simulink model "model_fully_coupled"  (R2021a)
settings: Solver=ode4  StartTime=0.0  StopTime=4  FixedStep=1e-2  RelTol=1e-3
values from neighbouring files (symbols this model uses):
  C_1 = [0.7887 -0.2113 -0.5774; -0.2113 0.7887 -0.5774; 0.5774 0.5774 0.5774]    [parameter.m]
  C_2 = [-0.2113 -0.5774 0.7887; 0.7887 -0.5774 -0.2113; 0.5774 0.5774 0.5774]    [parameter.m]
  C_3 = [-0.5774 0.7887 -0.2113; -0.5774 -0.2113 0.7887; 0.5774 0.5774 0.5774]    [parameter.m]
  d_1 = d    (= 4e-07)    [parameter.m]
  d_2 = d    (= 4e-07)    [parameter.m]
  d_3 = d    (= 4e-07)    [parameter.m]
  F = [0;0;0]    [parameter.m]
  g_s_1 = C_1(1:3,1)    [parameter.m]
  g_s_2 = C_2(1:3,1)    [parameter.m]
  g_s_3 = C_3(1:3,1)    [parameter.m]
  I = [1 0 0;0 1 0;0 0 1]    [parameter.m]
  I_hub_Bc = [550 0.1045 -0.0840; 0.1045 650 0.0001; -0.0840 0.0001 650]    [parameter.m]
  I_rw1_Wc1 = [1.5915E-4 0 1.54E-10; 0 0.8594E-4 0; 1.54E-10 0 0.8594E-4]    [parameter.m]
  I_rw1_Wc1_ = [0 -J_13_1 J_12_1; -J_13_1 (-2*J_23_1) (J_22_1-J_33_1); J_12_1 (J_22_1-J_33_1) (-2*J_23_1)]    [parameter.m]
  I_rw2_Wc2 = [1.5915E-4 0 1.54E-10; 0 0.8594E-4 0; 1.54E-10 0 0.8594E-4]    [parameter.m]
  I_rw2_Wc2_ = [0 -J_13_2 J_12_2; -J_13_2 (-2*J_23_2) (J_22_2-J_33_2); J_12_2 (J_22_2-J_33_2) (-2*J_23_2)]    [parameter.m]
  I_rw3_Wc3 = [1.5915E-4 0 1.54E-10; 0 0.8594E-4 0; 1.54E-10 0 0.8594E-4]    [parameter.m]
  I_rw3_Wc3_ = [0 -J_13_3 J_12_3; -J_13_3 (-2*J_23_3) (J_22_3-J_33_3); J_12_3 (J_22_3-J_33_3) (-2*J_23_3)]    [parameter.m]
  J_11_1 = I_rw1_Wc1(1,1)    [parameter.m]
  J_11_2 = I_rw2_Wc2(1,1)    [parameter.m]
  J_11_3 = I_rw3_Wc3(1,1)    [parameter.m]
  J_12_1 = I_rw1_Wc1(1,2)    [parameter.m]
  J_12_2 = I_rw2_Wc2(1,2)    [parameter.m]
  J_12_3 = I_rw3_Wc3(1,2)    [parameter.m]
  J_13_1 = I_rw1_Wc1(1,3)    [parameter.m]
  J_13_2 = I_rw2_Wc2(1,3)    [parameter.m]
  J_13_3 = I_rw3_Wc3(1,3)    [parameter.m]
  J_22_1 = I_rw1_Wc1(2,2)    [parameter.m]
  J_22_2 = I_rw2_Wc2(2,2)    [parameter.m]
  J_22_3 = I_rw3_Wc3(2,2)    [parameter.m]
  J_23_1 = I_rw1_Wc1(2,3)    [parameter.m]
  J_23_2 = I_rw2_Wc2(2,3)    [parameter.m]
  J_23_3 = I_rw3_Wc3(2,3)    [parameter.m]
  J_33_1 = I_rw1_Wc1(3,3)    [parameter.m]
  J_33_2 = I_rw2_Wc2(3,3)    [parameter.m]
  J_33_3 = I_rw3_Wc3(3,3)    [parameter.m]
  m_hub = 644    [parameter.m]
  m_rw_1 = m_rw(1)    [parameter.m]
  m_rw_2 = m_rw(2)    [parameter.m]
  m_rw_3 = m_rw(3)    [parameter.m]
  m_sc = 680    [parameter.m]
  OMEGA_1 = OMEGA(1)    [parameter.m]
  OMEGA_2 = OMEGA(2)    [parameter.m]
  OMEGA_3 = OMEGA(3)    [parameter.m]
  omega_BN = [omega ; omega; omega]    [parameter.m]
  r_Bc_B = [1e-2; -2e-2; 10e-2]    [parameter.m]
  r_BN = [0;0;0]    [parameter.m]
  r_W1_B = [0.6309; -0.1691; 0.4619]    [parameter.m]
  r_W2_B = [-0.1691; 0.6309; 0.4619]    [parameter.m]
  r_W3_B = [-0.4619; -0.4619; 0.4619]    [parameter.m]
  sigma_BN = [sigma; sigma; sigma]    [parameter.m]
  u_s_1 = u_s(1)    [parameter.m]
  u_s_2 = u_s(2)    [parameter.m]
  u_s_3 = u_s(3)    [parameter.m]
  w_2_1 = C_1(1:3,2)    [parameter.m]
  w_2_2 = C_2(1:3,2)    [parameter.m]
  w_2_3 = C_3(1:3,2)    [parameter.m]
  w_3_1 = C_1(1:3,3)    [parameter.m]
  w_3_2 = C_2(1:3,3)    [parameter.m]
  w_3_3 = C_3(1:3,3)    [parameter.m]
undefined symbols (not defined in the file or in its folder): deg, magnitude, rad, s
libraries: aerolibconvert2 x4, sharedutil x1, aerolibutil x1
(part 1 of 3)
settings Model: Creator=user  LastModifiedBy=user
settings DebuggingCC: AlgebraicLoopMsg=none

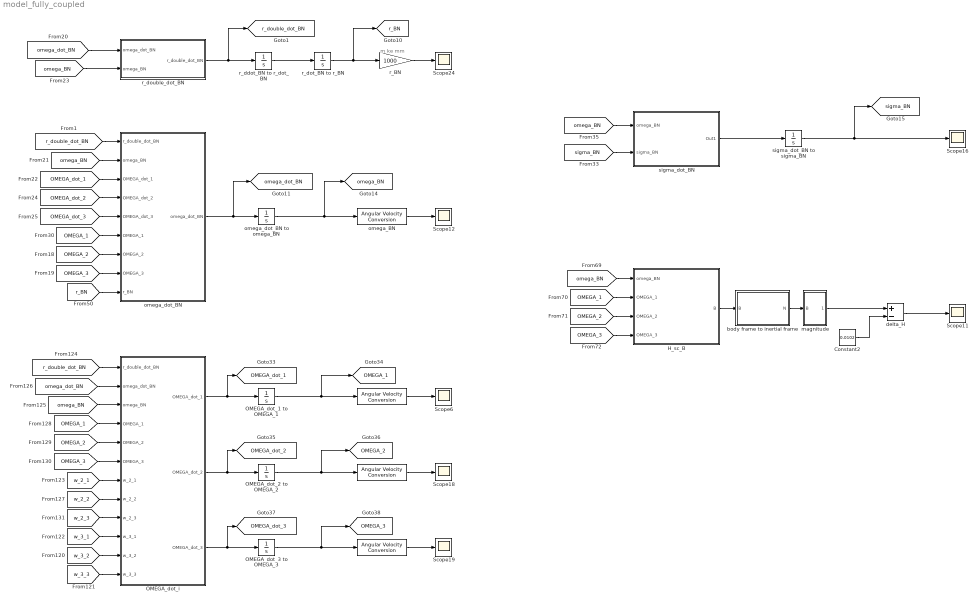
== system model_fully_coupled ==
  note: m ke mm
  " " : aerolibconvert2/Angular Velocity Conversion  IU=rad/s  OU=rpm
  "  " : aerolibconvert2/Angular Velocity Conversion  IU=rad/s  OU=rpm
  "   " : aerolibconvert2/Angular Velocity Conversion  IU=rad/s  OU=rpm
  Constant2 : Constant  Value=0.0102
  H_sc_B : Subsystem
  OMEGA_dot_1 to OMEGA_1 : Integrator  InitialCondition=OMEGA_1
  OMEGA_dot_2 to OMEGA_2 : Integrator  InitialCondition=OMEGA_2
  OMEGA_dot_3 to OMEGA_3 : Integrator  InitialCondition=OMEGA_3
  OMEGA_dot_i : Subsystem
  Scope{6,11..12,16,18..19,24} (7 alike) : Scope
  body frame to inertial frame : Subsystem
  delta_H : Sum  Inputs=+-
  magnitude : Subsystem
  omega_BN : aerolibconvert2/Angular Velocity Conversion  IU=rad/s  OU=deg/s
  omega_dot_BN : Subsystem
  omega_dot_BN to omega_BN : Integrator  InitialCondition=omega_BN
  r_BN : Gain  Gain=1000
  r_ddot_BN to r_dot_BN : Integrator  InitialCondition=r_BN
  r_dot_BN to r_BN : Integrator  InitialCondition=r_BN
  r_double_dot_BN : Subsystem
  sigma_dot_BN : Subsystem
  sigma_dot_BN to sigma_BN : Integrator  InitialCondition=sigma_BN
  tag scope: OMEGA_1=global, OMEGA_2=global, OMEGA_3=global, OMEGA_dot_1=global, OMEGA_dot_2=global, OMEGA_dot_3=global, omega_BN=global, omega_dot_BN=global, r_BN=global, r_double_dot_BN=global, sigma_BN=global
  wires:
  magnitude/1(Out1) -> delta_H/1
  [OMEGA_2] -> H_sc_B/3(OMEGA_2)
  H_sc_B/1(B) -> body frame to inertial frame/1(B)
  delta_H/1 -> Scope11/1
  [OMEGA_3] -> H_sc_B/4(OMEGA_3)
  [omega_BN] -> H_sc_B/1(omega_BN)
  [OMEGA_1] -> H_sc_B/2(OMEGA_1)
  Constant2/1 -> delta_H/2
  body frame to inertial frame/1(N) -> magnitude/1(B)
  r_dot_BN to r_BN/1 -> r_BN/1, [r_BN]
  r_double_dot_BN/1(r_double_dot_BN) -> [r_double_dot_BN], r_ddot_BN to r_dot_BN/1
  [omega_BN] -> r_double_dot_BN/2(omega_BN)
  r_ddot_BN to r_dot_BN/1 -> r_dot_BN to r_BN/1
  [omega_dot_BN] -> r_double_dot_BN/1(omega_dot_BN)
  r_BN/1 -> Scope24/1
  OMEGA_dot_2 to OMEGA_2/1 -> "  "/1, [OMEGA_2]
  [w_2_3] -> OMEGA_dot_i/9(w_2_3)
  [w_3_3] -> OMEGA_dot_i/12(w_3_3)
  [w_2_1] -> OMEGA_dot_i/7(w_2_1)
  OMEGA_dot_1 to OMEGA_1/1 -> [OMEGA_1], "   "/1
  [w_2_2] -> OMEGA_dot_i/8(w_2_2)
  OMEGA_dot_i/1(OMEGA_dot_1) -> OMEGA_dot_1 to OMEGA_1/1, [OMEGA_dot_1]
  [OMEGA_1] -> OMEGA_dot_i/4(OMEGA_1)
  OMEGA_dot_i/3(OMEGA_dot_3) -> [OMEGA_dot_3], OMEGA_dot_3 to OMEGA_3/1
  OMEGA_dot_i/2(OMEGA_dot_2) -> OMEGA_dot_2 to OMEGA_2/1, [OMEGA_dot_2]
  [omega_dot_BN] -> OMEGA_dot_i/2(omega_dot_BN)
  [omega_BN] -> OMEGA_dot_i/3(omega_BN)
  [r_double_dot_BN] -> OMEGA_dot_i/1(r_double_dot_BN)
  [OMEGA_2] -> OMEGA_dot_i/5(OMEGA_2)
  [w_3_2] -> OMEGA_dot_i/11(w_3_2)
  OMEGA_dot_3 to OMEGA_3/1 -> " "/1, [OMEGA_3]
  "   "/1 -> Scope6/1
  "  "/1 -> Scope18/1
  [w_3_1] -> OMEGA_dot_i/10(w_3_1)
  " "/1 -> Scope19/1
  [OMEGA_3] -> OMEGA_dot_i/6(OMEGA_3)
  [OMEGA_dot_2] -> omega_dot_BN/4(OMEGA_dot_2)
  omega_BN/1 -> Scope12/1
  omega_dot_BN to omega_BN/1 -> omega_BN/1, [omega_BN]
  [OMEGA_2] -> omega_dot_BN/7(OMEGA_2)
  [OMEGA_dot_3] -> omega_dot_BN/5(OMEGA_dot_3)
  [r_BN] -> omega_dot_BN/9(r_BN)
  [OMEGA_dot_1] -> omega_dot_BN/3(OMEGA_dot_1)
  [OMEGA_3] -> omega_dot_BN/8(OMEGA_3)
  [OMEGA_1] -> omega_dot_BN/6(OMEGA_1)
  omega_dot_BN/1("omega_dot_BN ") -> [omega_dot_BN], omega_dot_BN to omega_BN/1
  [omega_BN] -> omega_dot_BN/2(omega_BN)
  sigma_dot_BN/1(Out1) -> sigma_dot_BN to sigma_BN/1
  sigma_dot_BN to sigma_BN/1 -> Scope16/1, [sigma_BN]
  [sigma_BN] -> sigma_dot_BN/2(sigma_BN)
  [omega_BN] -> sigma_dot_BN/1(omega_BN)
  [r_double_dot_BN] -> omega_dot_BN/1(r_double_dot_BN)

== system model_fully_coupled/H_sc_B ==
  omega_BN : Inport
  OMEGA_1 : Inport  Port=2
  OMEGA_2 : Inport  Port=3
  OMEGA_3 : Inport  Port=4
  1 : Subsystem
  2 : Subsystem
  Add : Sum
  B : Outport
  wires:
  omega_BN/1 -> 2/1(omega_BN), 1/1(omega_BN)
  1/1(Out1) -> Add/1
  OMEGA_2/1 -> 2/3(OMEGA_2)
  OMEGA_3/1 -> 2/4(OMEGA_3)
  2/1(Out1) -> Add/2
  Add/1 -> B/1
  OMEGA_1/1 -> 2/2(OMEGA_1)

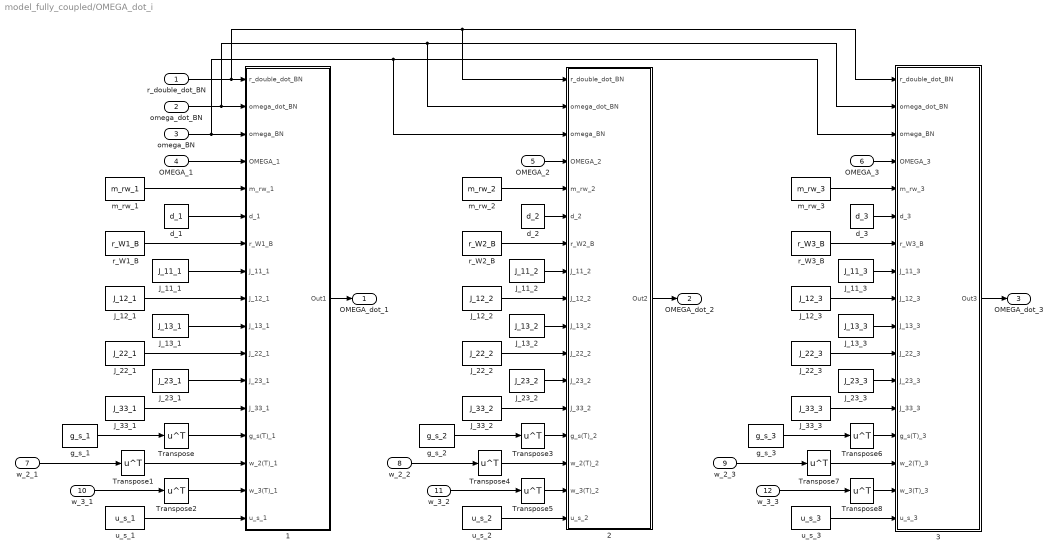
== system model_fully_coupled/OMEGA_dot_i ==
  r_double_dot_BN : Inport
  omega_dot_BN : Inport  Port=2
  omega_BN : Inport  Port=3
  OMEGA_1 : Inport  Port=4
  OMEGA_2 : Inport  Port=5
  OMEGA_3 : Inport  Port=6
  w_2_1 : Inport  Port=7
  w_2_2 : Inport  Port=8
  w_2_3 : Inport  Port=9
  w_3_1 : Inport  Port=10
  w_3_2 : Inport  Port=11
  w_3_3 : Inport  Port=12
  1 : Subsystem
  2 : Subsystem
  3 : Subsystem
  J_11_1 : Constant  Value=J_11_1
  J_11_2 : Constant  Value=J_11_2
  J_11_3 : Constant  Value=J_11_3
  J_12_1 : Constant  Value=J_12_1
  J_12_2 : Constant  Value=J_12_2
  J_12_3 : Constant  Value=J_12_3
  J_13_1 : Constant  Value=J_13_1
  J_13_2 : Constant  Value=J_13_2
  J_13_3 : Constant  Value=J_13_3
  J_22_1 : Constant  Value=J_22_1
  J_22_2 : Constant  Value=J_22_2
  J_22_3 : Constant  Value=J_22_3
  J_23_1 : Constant  Value=J_23_1
  J_23_2 : Constant  Value=J_23_2
  J_23_3 : Constant  Value=J_23_3
  J_33_1 : Constant  Value=J_33_1
  J_33_2 : Constant  Value=J_33_2
  J_33_3 : Constant  Value=J_33_3
  Transpose{,1..8} (9 alike) : Math  Operator=transpose  SaturateOnIntegerOverflow=on
  d_1 : Constant  Value=d_1
  d_2 : Constant  Value=d_2
  d_3 : Constant  Value=d_3
  g_s_1 : Constant  Value=g_s_1
  g_s_2 : Constant  Value=g_s_2
  g_s_3 : Constant  Value=g_s_3
  m_rw_1 : Constant  Value=m_rw_1
  m_rw_2 : Constant  Value=m_rw_2
  m_rw_3 : Constant  Value=m_rw_3
  r_W1_B : Constant  Value=r_W1_B
  r_W2_B : Constant  Value=r_W2_B
  r_W3_B : Constant  Value=r_W3_B
  u_s_1 : Constant  Value=u_s_1
  u_s_2 : Constant  Value=u_s_2
  u_s_3 : Constant  Value=u_s_3
  OMEGA_dot_1 : Outport
  OMEGA_dot_2 : Outport  Port=2
  OMEGA_dot_3 : Outport  Port=3
  wires:
  Transpose1/1 -> 1/15(w_2(T)_1)
  omega_dot_BN/1 -> 2/2(omega_dot_BN), 3/2(omega_dot_BN), 1/2(omega_dot_BN)
  w_3_1/1 -> Transpose2/1
  r_double_dot_BN/1 -> 2/1(r_double_dot_BN), 3/1(r_double_dot_BN), 1/1(r_double_dot_BN)
  g_s_1/1 -> Transpose/1
  J_23_1/1 -> 1/12(J_23_1)
  2/1(Out2) -> OMEGA_dot_2/1
  1/1(Out1) -> OMEGA_dot_1/1
  d_1/1 -> 1/6(d_1)
  m_rw_1/1 -> 1/5(m_rw_1)
  Transpose/1 -> 1/14(g_s(T)_1)
  J_33_1/1 -> 1/13(J_33_1)
  J_12_1/1 -> 1/9(J_12_1)
  omega_BN/1 -> 3/3(omega_BN), 2/3(omega_BN), 1/3(omega_BN)
  u_s_1/1 -> 1/17(u_s_1)
  Transpose2/1 -> 1/16(w_3(T)_1)
  3/1(Out3) -> OMEGA_dot_3/1
  J_11_1/1 -> 1/8(J_11_1)
  J_22_1/1 -> 1/11(J_22_1)
  J_13_1/1 -> 1/10(J_13_1)
  r_W1_B/1 -> 1/7(r_W1_B)
  w_2_1/1 -> Transpose1/1
  g_s_2/1 -> Transpose3/1
  J_23_2/1 -> 2/12(J_23_2)
  w_3_2/1 -> Transpose5/1
  r_W2_B/1 -> 2/7(r_W2_B)
  J_22_2/1 -> 2/11(J_22_2)
  J_11_2/1 -> 2/8(J_11_2)
  u_s_2/1 -> 2/17(u_s_2)
  J_12_2/1 -> 2/9(J_12_2)
  w_2_2/1 -> Transpose4/1
  Transpose3/1 -> 2/14(g_s(T)_2)
  m_rw_2/1 -> 2/5(m_rw_2)
  Transpose5/1 -> 2/16(w_3(T)_2)
  d_2/1 -> 2/6(d_2)
  J_33_2/1 -> 2/13(J_33_2)
  J_13_2/1 -> 2/10(J_13_2)
  Transpose4/1 -> 2/15(w_2(T)_2)
  g_s_3/1 -> Transpose6/1
  J_23_3/1 -> 3/12(J_23_3)
  w_3_3/1 -> Transpose8/1
  r_W3_B/1 -> 3/7(r_W3_B)
  J_22_3/1 -> 3/11(J_22_3)
  J_11_3/1 -> 3/8(J_11_3)
  u_s_3/1 -> 3/17(u_s_3)
  J_12_3/1 -> 3/9(J_12_3)
  w_2_3/1 -> Transpose7/1
  Transpose6/1 -> 3/14(g_s(T)_3)
  m_rw_3/1 -> 3/5(m_rw_3)
  Transpose8/1 -> 3/16(w_3(T)_3)
  d_3/1 -> 3/6(d_3)
  J_33_3/1 -> 3/13(J_33_3)
  J_13_3/1 -> 3/10(J_13_3)
  Transpose7/1 -> 3/15(w_2(T)_3)
  OMEGA_1/1 -> 1/4(OMEGA_1)
  OMEGA_2/1 -> 2/4(OMEGA_2)
  OMEGA_3/1 -> 3/4(OMEGA_3)

== system model_fully_coupled/body frame to inertial frame ==
  B : Inport
  MATLAB Function : MATLAB Function  TreatAsAtomicUnit=on
  N : Outport
  wires:
  MATLAB Function/1(N) -> N/1
  B/1 -> MATLAB Function/1(B)
  [sigma_BN] -> MATLAB Function/2(sigma_BN)

== system model_fully_coupled/magnitude ==
  B : Inport
  Add : Sum  Inputs=+++
  Demux : Demux  Outputs=3
  Magnitude Squared : Math  Operator=magnitude^2  SaturateOnIntegerOverflow=on
  Magnitude Squared1 : Math  Operator=magnitude^2  SaturateOnIntegerOverflow=on
  Magnitude Squared2 : Math  Operator=magnitude^2  SaturateOnIntegerOverflow=on
  Sqrt : Sqrt  SaturateOnIntegerOverflow=on
  Out1 : Outport
  wires:
  Add/1 -> Sqrt/1
  B/1 -> Demux/1
  Sqrt/1 -> Out1/1
  Demux/1 -> Magnitude Squared/1
  Demux/2 -> Magnitude Squared1/1
  Demux/3 -> Magnitude Squared2/1
  Magnitude Squared1/1 -> Add/2
  Magnitude Squared/1 -> Add/1
  Magnitude Squared2/1 -> Add/3

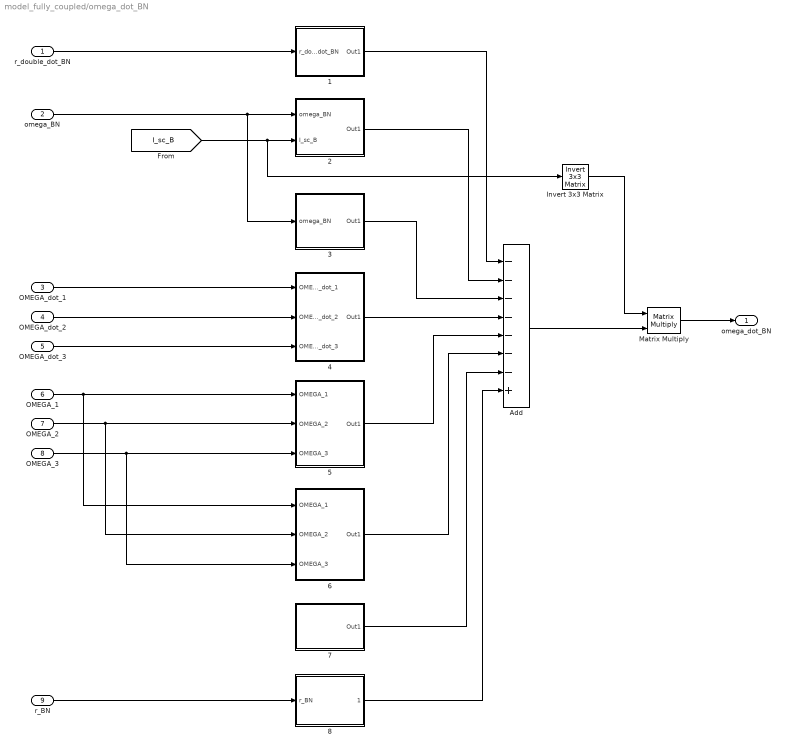
== system model_fully_coupled/omega_dot_BN ==
  r_double_dot_BN : Inport
  omega_BN : Inport  Port=2
  OMEGA_dot_1 : Inport  Port=3
  OMEGA_dot_2 : Inport  Port=4
  OMEGA_dot_3 : Inport  Port=5
  OMEGA_1 : Inport  Port=6
  OMEGA_2 : Inport  Port=7
  OMEGA_3 : Inport  Port=8
  r_BN : Inport  Port=9
  1 : Subsystem
  "2 " : Subsystem
  3 : Subsystem
  4 : Subsystem
  5 : Subsystem
  6 : Subsystem
  "7 " : Subsystem
  8 : Subsystem
  Add : Sum  Inputs=-------+
  Invert 3x3 Matrix : aerolibutil/Invert  3x3 Matrix
  Matrix Multiply : Product  Multiplication=Matrix(*)
  "omega_dot_BN " : Outport
  wires:
  OMEGA_2/1 -> 6/2(OMEGA_2), 5/2(OMEGA_2)
  OMEGA_dot_3/1 -> 4/3(OMEGA_dot_3)
  OMEGA_1/1 -> 6/1(OMEGA_1), 5/1(OMEGA_1)
  OMEGA_dot_1/1 -> 4/1(OMEGA_dot_1)
  omega_BN/1 -> 3/1(omega_BN), "2 "/1(omega_BN)
  OMEGA_dot_2/1 -> 4/2(OMEGA_dot_2)
  OMEGA_3/1 -> 6/3(OMEGA_3), 5/3(OMEGA_3)
  Matrix Multiply/1 -> "omega_dot_BN "/1
  Add/1 -> Matrix Multiply/2
  Invert 3x3 Matrix/1 -> Matrix Multiply/1
  [I_sc_B] -> Invert 3x3 Matrix/1, "2 "/2(I_sc_B)
  r_BN/1 -> 8/1(r_BN)
  1/1(Out1) -> Add/1
  "2 "/1(Out1) -> Add/2
  3/1(Out1) -> Add/3
  4/1(Out1) -> Add/4
  5/1(Out1) -> Add/5
  6/1(Out1) -> Add/6
  "7 "/1(Out1) -> Add/7
  8/1(1) -> Add/8
  r_double_dot_BN/1 -> 1/1(r_double_dot_BN)

== system model_fully_coupled/r_double_dot_BN ==
  omega_dot_BN : Inport
  omega_BN : Inport  Port=2
  Add : Sum  Inputs=+-
  c_double_dot : Subsystem
  r_double_dot_CN : Subsystem
  r_double_dot_BN : Outport
  wires:
  c_double_dot/1(Out1) -> Add/2
  r_double_dot_CN/1(Out1) -> Add/1
  omega_BN/1 -> c_double_dot/2(omega_BN)
  omega_dot_BN/1 -> c_double_dot/1(omega_dot_BN)
  Add/1 -> r_double_dot_BN/1

== system model_fully_coupled/sigma_dot_BN ==
  omega_BN : Inport
  sigma_BN : Inport  Port=2
  Add : Sum  Inputs=+-
  Add1 : Sum  Inputs=+-+
  Constant : Constant
  Matrix Multiply1 : Product  Multiplication=Matrix(*)
  Matrix Multiply2 : Product  Multiplication=Matrix(*)
  Matrix Multiply3 : Product  Multiplication=Matrix(*)
  Multiply : Gain  Gain=I/2
  Multiply1 : Gain  Gain=1/2
  Subsystem : Subsystem
  Transpose : Math  Operator=transpose  SaturateOnIntegerOverflow=on
  Out1 : Outport
  wires:
  Add1/1 -> Multiply1/1
  Subsystem/1("skew ") -> Add1/2
  Matrix Multiply2/1 -> Add1/3
  Transpose/1 -> Matrix Multiply2/2, Matrix Multiply1/1
  sigma_BN/1 -> Transpose/1, Matrix Multiply1/2, Matrix Multiply2/1, Subsystem/1(sigma_BN)
  Matrix Multiply1/1 -> Add/2
  Add/1 -> Multiply/1
  Constant/1 -> Add/1
  Multiply/1 -> Add1/1
  Multiply1/1 -> Matrix Multiply3/1
  omega_BN/1 -> Matrix Multiply3/2
  Matrix Multiply3/1 -> Out1/1

== system model_fully_coupled/H_sc_B/1 ==
  omega_BN : Inport
  Add : Sum
  Constant : Constant  Value=I_hub_Bc
  Constant1 : Constant  Value=r_Bc_B
  Constant2 : Constant  Value=m_hub
  Integrator1 : Integrator  InitialConditionSource=external
  Matrix Multiply : Product  Multiplication=Matrix(*)
  Matrix Multiply1 : Product  Multiplication=Matrix(*)
  Product : Product
  Scope : Scope
  Scope1 : Scope
  Subsystem : Subsystem
  Subsystem1 : Subsystem
  Out1 : Outport
  tag scope: r_Bc_B=global, r_Bc_B_skew=global
  wires:
  omega_BN/1 -> Matrix Multiply/2
  Constant/1 -> Matrix Multiply/1
  Subsystem/1(Out1) -> Matrix Multiply1/2, Integrator1/1
  Constant1/1 -> Integrator1/2
  Integrator1/1 -> [r_Bc_B], Subsystem1/1(1)
  Subsystem1/1("skew ") -> [r_Bc_B_skew], Matrix Multiply1/1
  Matrix Multiply1/1 -> Product/2
  Constant2/1 -> Product/1
  Matrix Multiply/1 -> Scope1/1, Add/1
  Product/1 -> Scope/1, Add/2
  Add/1 -> Out1/1

== system model_fully_coupled/H_sc_B/2 ==
  omega_BN : Inport
  OMEGA_1 : Inport  Port=2
  OMEGA_2 : Inport  Port=3
  OMEGA_3 : Inport  Port=4
  Add : Sum  Inputs=+++
  H_rw1_B : Subsystem
  H_rw2_B : Subsystem
  H_rw3_B : Subsystem
  I_rwi_Wci1 : Subsystem
  Subsystem : Subsystem
  d_i : Subsystem
  g_s_i : Subsystem
  Out1 : Outport
  wires:
  omega_BN/1 -> H_rw3_B/5(omega_BN), H_rw2_B/5(omega_BN), H_rw1_B/5(omega_BN)
  OMEGA_1/1 -> H_rw1_B/6(OMEGA_1)
  OMEGA_2/1 -> H_rw2_B/6(OMEGA_2)
  OMEGA_3/1 -> H_rw3_B/6(OMEGA_3)
  I_rwi_Wci1/1(Out1) -> H_rw1_B/1(I_rw1_Wc1)
  g_s_i/1(Out1) -> H_rw1_B/2(g_s_1)
  I_rwi_Wci1/2(2) -> H_rw2_B/1(I_rw2_Wc2)
  I_rwi_Wci1/3(3) -> H_rw3_B/1(I_rw3_Wc3)
  g_s_i/2(Out2) -> H_rw2_B/2(g_s_2)
  g_s_i/3(Out3) -> H_rw3_B/2(g_s_3)
  H_rw2_B/1(Out1) -> Add/2
  Add/1 -> Out1/1
  H_rw1_B/1(Out1) -> Add/1
  H_rw3_B/1(Out1) -> Add/3
  d_i/1(1) -> H_rw1_B/3(d_1)
  d_i/2(Out3) -> H_rw2_B/3(d_2)
  d_i/3(Out2) -> H_rw3_B/3(d_3)
  Subsystem/1(w_3_1) -> H_rw1_B/4(w_3_1)
  Subsystem/2(w_3_2) -> H_rw2_B/4(w_3_2)
  Subsystem/3(w_3_3) -> H_rw3_B/4(w_3_3)

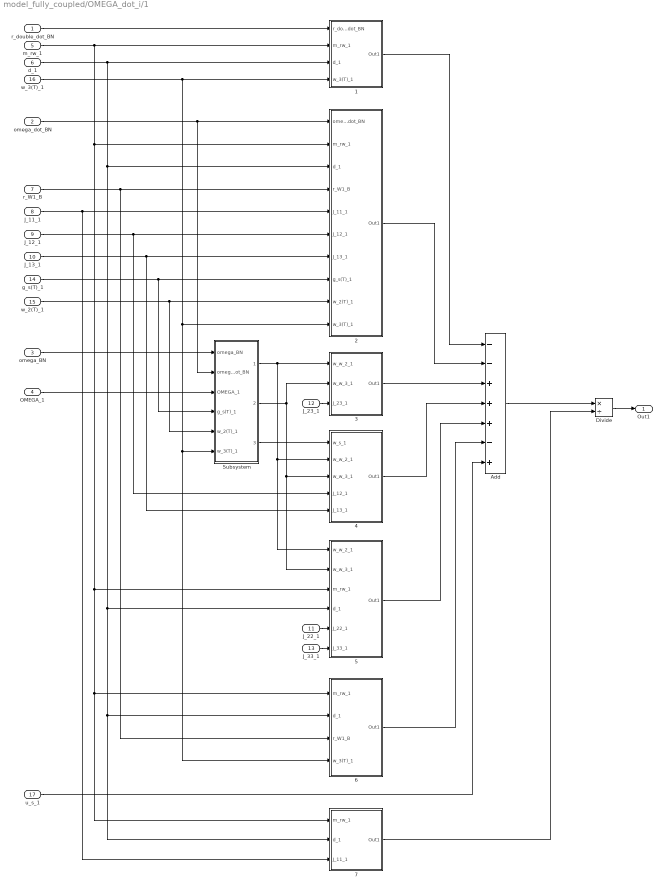
== system model_fully_coupled/OMEGA_dot_i/1 ==
  r_double_dot_BN : Inport
  omega_dot_BN : Inport  Port=2
  omega_BN : Inport  Port=3
  OMEGA_1 : Inport  Port=4
  m_rw_1 : Inport  Port=5
  d_1 : Inport  Port=6
  r_W1_B : Inport  Port=7
  J_11_1 : Inport  Port=8
  J_12_1 : Inport  Port=9
  J_13_1 : Inport  Port=10
  J_22_1 : Inport  Port=11
  J_23_1 : Inport  Port=12
  J_33_1 : Inport  Port=13
  g_s(T)_1 : Inport  Port=14
  w_2(T)_1 : Inport  Port=15
  w_3(T)_1 : Inport  Port=16
  u_s_1 : Inport  Port=17
  1 : Subsystem
  2 : Subsystem
  3 : Subsystem
  4 : Subsystem
  5 : Subsystem
  6 : Subsystem
  7 : Subsystem
  Add : Sum  Inputs=--+++-+
  Divide : Product  Inputs=*/
  Subsystem : Subsystem
  Out1 : Outport
  wires:
  Subsystem/2(2) -> 5/2(w_w_3_1), 4/3(w_w_3_1), 3/2(w_w_3_1)
  r_double_dot_BN/1 -> 1/1(r_double_dot_BN)
  J_23_1/1 -> 3/3(J_23_1)
  r_W1_B/1 -> 6/3(r_W1_B), 2/4(r_W1_B)
  omega_dot_BN/1 -> Subsystem/2(omega_dot_BN), 2/1(omega_dot_BN)
  J_12_1/1 -> 4/4(J_12_1), 2/6(J_12_1)
  J_22_1/1 -> 5/5(J_22_1)
  J_11_1/1 -> 7/3(J_11_1), 2/5(J_11_1)
  d_1/1 -> 2/3(d_1), 7/2(d_1), 6/2(d_1), 5/4(d_1), 1/3(d_1)
  w_3(T)_1/1 -> 6/4(w_3(T)_1), Subsystem/6(w_3(T)_1), 2/10(w_3(T)_1), 1/4(w_3(T)_1)
  m_rw_1/1 -> 1/2(m_rw_1), 2/2(m_rw_1), 7/1(m_rw_1), 6/1(m_rw_1), 5/3(m_rw_1)
  J_33_1/1 -> 5/6(J_33_1)
  g_s(T)_1/1 -> 2/8(g_s(T)_1), Subsystem/4(g_s(T)_1)
  J_13_1/1 -> 4/5(J_13_1), 2/7(J_13_1)
  w_2(T)_1/1 -> 2/9(w_2(T)_1), Subsystem/5(w_2(T)_1)
  3/1(Out1) -> Add/3
  2/1(Out1) -> Add/2
  1/1(Out1) -> Add/1
  4/1(Out1) -> Add/4
  5/1(Out1) -> Add/5
  6/1(Out1) -> Add/6
  u_s_1/1 -> Add/7
  Add/1 -> Divide/1
  7/1(Out1) -> Divide/2
  Divide/1 -> Out1/1
  Subsystem/1(1) -> 5/1(w_w_2_1), 4/2(w_w_2_1), 3/1(w_w_2_1)
  omega_BN/1 -> Subsystem/1(omega_BN)
  Subsystem/3(3) -> 4/1(w_s_1)
  OMEGA_1/1 -> Subsystem/3(OMEGA_1)

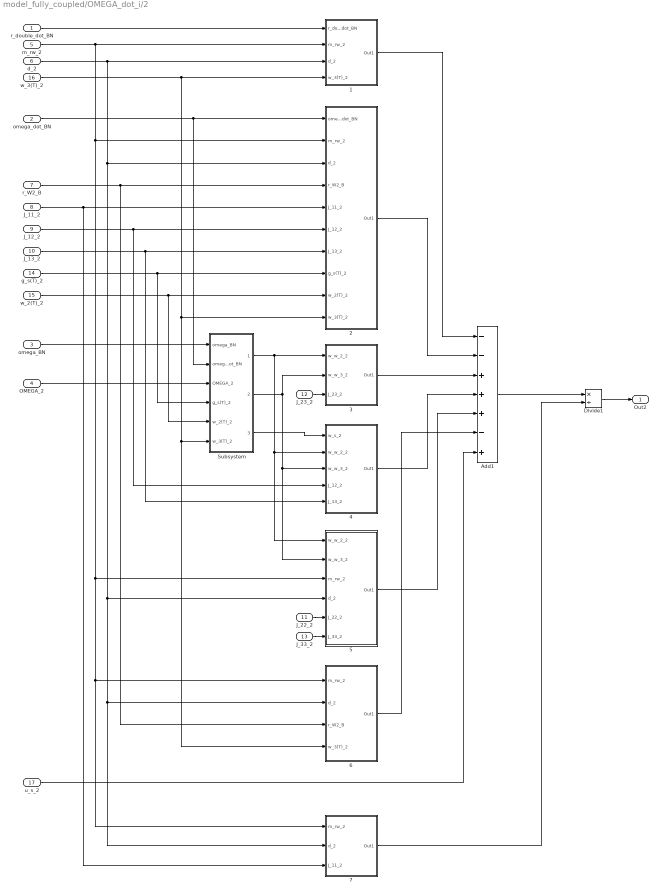
== system model_fully_coupled/OMEGA_dot_i/2 ==
  r_double_dot_BN : Inport
  omega_dot_BN : Inport  Port=2
  omega_BN : Inport  Port=3
  OMEGA_2 : Inport  Port=4
  m_rw_2 : Inport  Port=5
  d_2 : Inport  Port=6
  r_W2_B : Inport  Port=7
  J_11_2 : Inport  Port=8
  J_12_2 : Inport  Port=9
  J_13_2 : Inport  Port=10
  J_22_2 : Inport  Port=11
  J_23_2 : Inport  Port=12
  J_33_2 : Inport  Port=13
  g_s(T)_2 : Inport  Port=14
  w_2(T)_2 : Inport  Port=15
  w_3(T)_2 : Inport  Port=16
  u_s_2 : Inport  Port=17
  1 : Subsystem
  2 : Subsystem
  3 : Subsystem
  4 : Subsystem
  5 : Subsystem
  6 : Subsystem
  7 : Subsystem
  Add1 : Sum  Inputs=--+++-+
  Divide1 : Product  Inputs=*/
  Subsystem : Subsystem
  Out2 : Outport
  wires:
  3/1(Out1) -> Add1/3
  J_33_2/1 -> 5/6(J_33_2)
  d_2/1 -> 2/3(d_2), 7/2(d_2), 6/2(d_2), 5/4(d_2), 1/3(d_2)
  w_3(T)_2/1 -> Subsystem/6(w_3(T)_2), 6/4(w_3(T)_2), 2/10(w_3(T)_2), 1/4(w_3(T)_2)
  Add1/1 -> Divide1/1
  Divide1/1 -> Out2/1
  1/1(Out1) -> Add1/1
  m_rw_2/1 -> 1/2(m_rw_2), 2/2(m_rw_2), 7/1(m_rw_2), 6/1(m_rw_2), 5/3(m_rw_2)
  w_2(T)_2/1 -> Subsystem/5(w_2(T)_2), 2/9(w_2(T)_2)
  J_22_2/1 -> 5/5(J_22_2)
  J_12_2/1 -> 4/4(J_12_2), 2/6(J_12_2)
  r_double_dot_BN/1 -> 1/1(r_double_dot_BN)
  4/1(Out1) -> Add1/4
  g_s(T)_2/1 -> Subsystem/4(g_s(T)_2), 2/8(g_s(T)_2)
  J_23_2/1 -> 3/3(J_23_2)
  r_W2_B/1 -> 6/3(r_W2_B), 2/4(r_W2_B)
  Subsystem/3(3) -> 4/1(w_s_2)
  J_11_2/1 -> 7/3(J_11_2), 2/5(J_11_2)
  omega_dot_BN/1 -> Subsystem/2(omega_dot_BN), 2/1(omega_dot_BN)
  Subsystem/2(2) -> 5/2(w_w_3_2), 4/3(w_w_3_2), 3/2(w_w_3_2)
  u_s_2/1 -> Add1/7
  6/1(Out1) -> Add1/6
  7/1(Out1) -> Divide1/2
  5/1(Out1) -> Add1/5
  J_13_2/1 -> 4/5(J_13_2), 2/7(J_13_2)
  Subsystem/1(1) -> 5/1(w_w_2_2), 4/2(w_w_2_2), 3/1(w_w_2_2)
  2/1(Out1) -> Add1/2
  omega_BN/1 -> Subsystem/1(omega_BN)
  OMEGA_2/1 -> Subsystem/3(OMEGA_2)

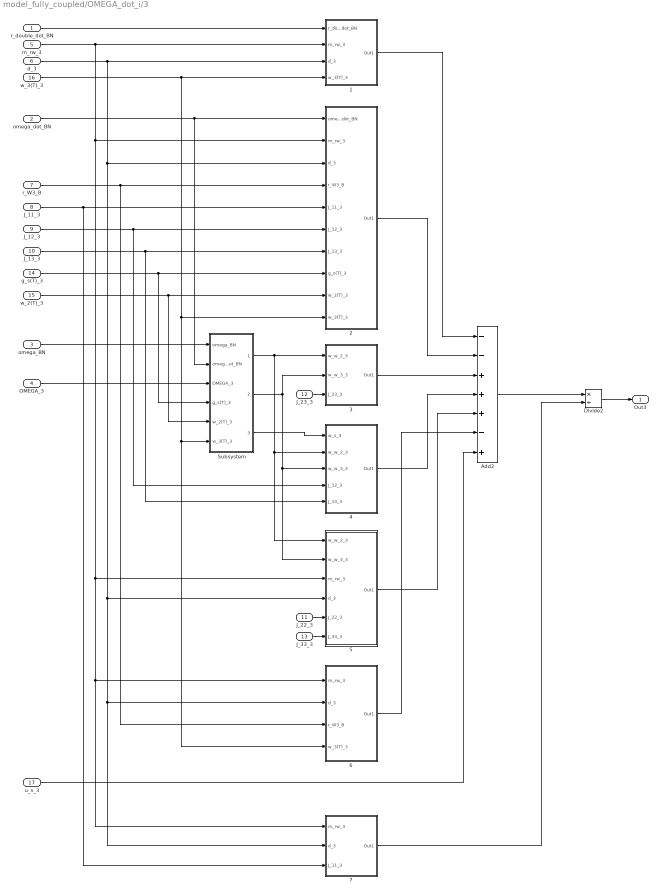
== system model_fully_coupled/OMEGA_dot_i/3 ==
  r_double_dot_BN : Inport
  omega_dot_BN : Inport  Port=2
  omega_BN : Inport  Port=3
  OMEGA_3 : Inport  Port=4
  m_rw_3 : Inport  Port=5
  d_3 : Inport  Port=6
  r_W3_B : Inport  Port=7
  J_11_3 : Inport  Port=8
  J_12_3 : Inport  Port=9
  J_13_3 : Inport  Port=10
  J_22_3 : Inport  Port=11
  J_23_3 : Inport  Port=12
  J_33_3 : Inport  Port=13
  g_s(T)_3 : Inport  Port=14
  w_2(T)_3 : Inport  Port=15
  w_3(T)_3 : Inport  Port=16
  u_s_3 : Inport  Port=17
  1 : Subsystem
  2 : Subsystem
  3 : Subsystem
  4 : Subsystem
  5 : Subsystem
  6 : Subsystem
  7 : Subsystem
  Add2 : Sum  Inputs=--+++-+
  Divide2 : Product  Inputs=*/
  Subsystem : Subsystem
  Out3 : Outport
  wires:
  Subsystem/1(1) -> 5/1(w_w_2_3), 4/2(w_w_2_3), 3/1(w_w_2_3)
  7/1(Out1) -> Divide2/2
  d_3/1 -> 2/3(d_3), 7/2(d_3), 6/2(d_3), 5/4(d_3), 1/3(d_3)
  6/1(Out1) -> Add2/6
  u_s_3/1 -> Add2/7
  r_W3_B/1 -> 6/3(r_W3_B), 2/4(r_W3_B)
  w_2(T)_3/1 -> Subsystem/5(w_2(T)_3), 2/9(w_2(T)_3)
  1/1(Out1) -> Add2/1
  2/1(Out1) -> Add2/2
  w_3(T)_3/1 -> Subsystem/6(w_3(T)_3), 6/4(w_3(T)_3), 2/10(w_3(T)_3), 1/4(w_3(T)_3)
  Divide2/1 -> Out3/1
  J_22_3/1 -> 5/5(J_22_3)
  4/1(Out1) -> Add2/4
  m_rw_3/1 -> 1/2(m_rw_3), 2/2(m_rw_3), 7/1(m_rw_3), 6/1(m_rw_3), 5/3(m_rw_3)
  J_33_3/1 -> 5/6(J_33_3)
  J_23_3/1 -> 3/3(J_23_3)
  J_12_3/1 -> 4/4(J_12_3), 2/6(J_12_3)
  g_s(T)_3/1 -> Subsystem/4(g_s(T)_3), 2/8(g_s(T)_3)
  J_11_3/1 -> 7/3(J_11_3), 2/5(J_11_3)
  omega_dot_BN/1 -> Subsystem/2(omega_dot_BN), 2/1(omega_dot_BN)
  Subsystem/3(3) -> 4/1(w_s_3)
  5/1(Out1) -> Add2/5
  r_double_dot_BN/1 -> 1/1(r_double_dot_BN)
  Subsystem/2(2) -> 5/2(w_w_3_3), 4/3(w_w_3_3), 3/2(w_w_3_3)
  J_13_3/1 -> 4/5(J_13_3), 2/7(J_13_3)
  Add2/1 -> Divide2/1
  3/1(Out1) -> Add2/3
  omega_BN/1 -> Subsystem/1(omega_BN)
  OMEGA_3/1 -> Subsystem/3(OMEGA_3)

== system model_fully_coupled/omega_dot_BN/1 ==
  r_double_dot_BN : Inport
  Matrix Multiply2 : Product  Multiplication=Matrix(*)
  Product : Product
  m_sc : Constant
  Out1 : Outport
  wires:
  r_double_dot_BN/1 -> Matrix Multiply2/2
  Product/1 -> Out1/1
  m_sc/1 -> Product/1
  Matrix Multiply2/1 -> Product/2
  [c_skew] -> Matrix Multiply2/1

== system model_fully_coupled/omega_dot_BN/2  ==
  omega_BN : Inport
  I_sc_B : Inport  Port=2
  Matrix Multiply : Product  Multiplication=Matrix(*)
  Matrix Multiply1 : Product  Multiplication=Matrix(*)
  Subsystem1 : Subsystem
  Out1 : Outport
  wires:
  omega_BN/1 -> Subsystem1/1(1), Matrix Multiply1/2
  Matrix Multiply1/1 -> Out1/1
  I_sc_B/1 -> Matrix Multiply/2
  Matrix Multiply/1 -> Matrix Multiply1/1
  Subsystem1/1("skew ") -> Matrix Multiply/1

== system model_fully_coupled/omega_dot_BN/3 ==
  omega_BN : Inport
  I_sc_B : Subsystem
  I_sc_B' : Subsystem
  Integrator : Integrator  InitialConditionSource=external
  Matrix Multiply3 : Product  Multiplication=Matrix(*)
  Out1 : Outport
  tag scope: I_sc_B=global
  wires:
  I_sc_B'/1(Out1) -> Matrix Multiply3/1, Integrator/1
  Matrix Multiply3/1 -> Out1/1
  omega_BN/1 -> Matrix Multiply3/2
  Integrator/1 -> [I_sc_B]
  I_sc_B/1(I_sc_B) -> Integrator/2
  [OMEGA_1] -> I_sc_B/1(OMEGA_1)
  [OMEGA_2] -> I_sc_B/2(OMEGA_2)
  [OMEGA_3] -> I_sc_B/3(OMEGA_3)

== system model_fully_coupled/omega_dot_BN/4 ==
  OMEGA_dot_1 : Inport
  OMEGA_dot_2 : Inport  Port=2
  OMEGA_dot_3 : Inport  Port=3
  Add : Sum  Inputs=+++
  I_rwi_Wci : Subsystem
  Matrix Multiply1 : Product  Multiplication=Matrix(*)
  Matrix Multiply3 : Product  Multiplication=Matrix(*)
  Matrix Multiply4 : Product  Multiplication=Matrix(*)
  Product3 : Product
  Product6 : Product
  Product9 : Product
  g_s_i : Subsystem
  Out1 : Outport
  wires:
  Product9/1 -> Add/3
  Product3/1 -> Add/1
  Product6/1 -> Add/2
  Add/1 -> Out1/1
  Matrix Multiply4/1 -> Product3/1
  OMEGA_dot_1/1 -> Product3/2
  I_rwi_Wci/1(Out1) -> Matrix Multiply4/1
  g_s_i/1(Out1) -> Matrix Multiply4/2
  Matrix Multiply1/1 -> Product6/1
  g_s_i/2(Out2) -> Matrix Multiply1/2
  I_rwi_Wci/2(Out2) -> Matrix Multiply1/1
  OMEGA_dot_2/1 -> Product6/2
  Matrix Multiply3/1 -> Product9/1
  OMEGA_dot_3/1 -> Product9/2
  I_rwi_Wci/3(Out3) -> Matrix Multiply3/1
  g_s_i/3(Out3) -> Matrix Multiply3/2

== system model_fully_coupled/omega_dot_BN/5 ==
  OMEGA_1 : Inport
  OMEGA_2 : Inport  Port=2
  OMEGA_3 : Inport  Port=3
  Add : Sum  Inputs=+++
  I_rwi_Wci' : Subsystem
  Matrix Multiply1 : Product  Multiplication=Matrix(*)
  Matrix Multiply2 : Product  Multiplication=Matrix(*)
  Matrix Multiply4 : Product  Multiplication=Matrix(*)
  Product1 : Product
  Product2 : Product
  Product3 : Product
  g_s_i : Subsystem
  Out1 : Outport
  wires:
  Matrix Multiply1/1 -> Add/2
  Matrix Multiply2/1 -> Add/3
  Matrix Multiply4/1 -> Add/1
  Add/1 -> Out1/1
  I_rwi_Wci'/1(Out1) -> Matrix Multiply4/1
  g_s_i/1(Out1) -> Product1/2
  OMEGA_1/1 -> Product1/1
  Product1/1 -> Matrix Multiply4/2
  Product2/1 -> Matrix Multiply1/2
  OMEGA_2/1 -> Product2/1
  I_rwi_Wci'/2(Out2) -> Matrix Multiply1/1
  g_s_i/2(Out2) -> Product2/2
  g_s_i/3(Out3) -> Product3/2
  Product3/1 -> Matrix Multiply2/2
  I_rwi_Wci'/3(Out3) -> Matrix Multiply2/1
  OMEGA_3/1 -> Product3/1

== system model_fully_coupled/omega_dot_BN/6 ==
  OMEGA_1 : Inport
  OMEGA_2 : Inport  Port=2
  OMEGA_3 : Inport  Port=3
  1 : Subsystem
  2 : Subsystem
  3 : Subsystem
  Add : Sum  Inputs=+++
  I_rwi_Wci : Subsystem
  Matrix Multiply4 : Product  Multiplication=Matrix(*)
  g_s_i : Subsystem
  m_rw_i : Subsystem
  Out1 : Outport
  wires:
  Add/1 -> Matrix Multiply4/2
  I_rwi_Wci/2(Out2) -> 2/1(I_rw2_Wc2)
  g_s_i/1(Out1) -> 1/2(g_s_1)
  m_rw_i/1(Out1) -> 1/3(m_rw_1)
  g_s_i/2(Out2) -> 2/2(g_s_2)
  [omega_BN_skew] -> Matrix Multiply4/1
  OMEGA_3/1 -> 3/4(OMEGA_3)
  m_rw_i/2(Out2) -> 2/3(m_rw_2)
  1/1(Out1) -> Add/1
  Matrix Multiply4/1 -> Out1/1
  OMEGA_1/1 -> 1/4(OMEGA_1)
  I_rwi_Wci/3(Out3) -> 3/1(I_rw3_Wc3)
  2/1(Out2) -> Add/2
  3/1(Out3) -> Add/3
  g_s_i/3(Out3) -> 3/2(g_s_3)
  I_rwi_Wci/1(Out1) -> 1/1(I_rw1_Wc1)
  m_rw_i/3(Out3) -> 3/3(m_rw_3)
  OMEGA_2/1 -> 2/4(OMEGA_2)

== system model_fully_coupled/omega_dot_BN/7  ==
  Add : Sum  Inputs=+++
  Matrix Multiply2 : Product  Multiplication=Matrix(*)
  Matrix Multiply5 : Product  Multiplication=Matrix(*)
  Matrix Multiply6 : Product  Multiplication=Matrix(*)
  Product2 : Product
  Product4 : Product
  Product6 : Product
  m_rw_i : Subsystem
  Out1 : Outport
  wires:
  Product2/1 -> Add/1
  Product6/1 -> Add/3
  Product4/1 -> Add/2
  Add/1 -> Out1/1
  [r_dprime_Wc1_B] -> Matrix Multiply5/2
  [r_Wc1_B_skew] -> Matrix Multiply5/1
  m_rw_i/1(Out1) -> Product2/1
  Matrix Multiply5/1 -> Product2/2
  [r_dprime_Wc2_B] -> Matrix Multiply2/2
  [r_Wc2_B_skew] -> Matrix Multiply2/1
  m_rw_i/2(Out2) -> Product4/1
  Matrix Multiply2/1 -> Product4/2
  [r_dprime_Wc3_B] -> Matrix Multiply6/2
  [r_Wc3_B_skew] -> Matrix Multiply6/1
  m_rw_i/3(Out3) -> Product6/1
  Matrix Multiply6/1 -> Product6/2

== system model_fully_coupled/omega_dot_BN/8 ==
  r_BN : Inport
  3x3 Cross Product : sharedutil/3x3 Cross Product  aMode=aMode
      settings: SourceProductBaseCode=AE,PW,DR,MT,UV,VE
  Add1 : Sum  Inputs=+-
  F : Constant  Value=F
  r_P : Constant  Value=0
  1 : Outport
  wires:
  3x3 Cross Product/1 -> 1/1
  F/1 -> 3x3 Cross Product/2
  Add1/1 -> 3x3 Cross Product/1
  r_P/1 -> Add1/2
  r_BN/1 -> Add1/1

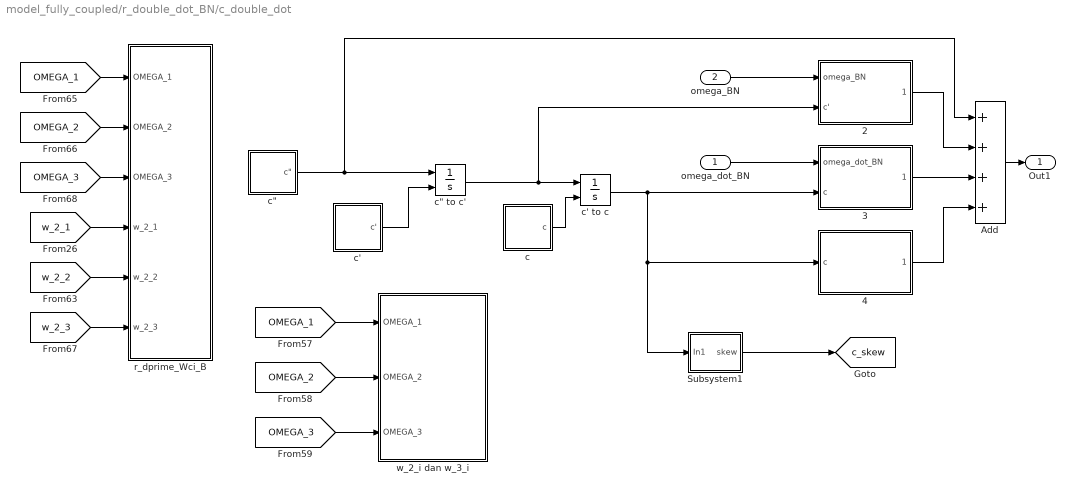
== system model_fully_coupled/r_double_dot_BN/c_double_dot ==
  omega_dot_BN : Inport
  omega_BN : Inport  Port=2
  2 : Subsystem
  3 : Subsystem
  4 : Subsystem
  Add : Sum  Inputs=++++
  Subsystem1 : Subsystem
  c : Subsystem
  "c\"" : Subsystem
  "c\" to c'" : Integrator  InitialConditionSource=external
  c' : Subsystem
  c' to c : Integrator  InitialConditionSource=external
  r_dprime_Wci_B : Subsystem
  w_2_i dan w_3_i : Subsystem
  Out1 : Outport
  tag scope: c_skew=global
  wires:
  c' to c/1 -> Subsystem1/1(In1), 4/1(c), 3/2(c)
  4/1(1) -> Add/4
  3/1(1) -> Add/3
  omega_dot_BN/1 -> 3/1(omega_dot_BN)
  "c\" to c'"/1 -> 2/2(c'), c' to c/1
  "c\""/1("c\"") -> Add/1, "c\" to c'"/1
  c'/1(c') -> "c\" to c'"/2
  2/1(1) -> Add/2
  c/1(c) -> c' to c/2
  Add/1 -> Out1/1
  omega_BN/1 -> 2/1(omega_BN)
  Subsystem1/1("skew ") -> [c_skew]
  [OMEGA_2] -> r_dprime_Wci_B/2(OMEGA_2)
  [w_2_3] -> r_dprime_Wci_B/6(w_2_3)
  [OMEGA_1] -> r_dprime_Wci_B/1(OMEGA_1)
  [w_2_1] -> r_dprime_Wci_B/4(w_2_1)
  [w_2_2] -> r_dprime_Wci_B/5(w_2_2)
  [OMEGA_3] -> r_dprime_Wci_B/3(OMEGA_3)
  [OMEGA_3] -> w_2_i dan w_3_i/3(OMEGA_3)
  [OMEGA_1] -> w_2_i dan w_3_i/1(OMEGA_1)
  [OMEGA_2] -> w_2_i dan w_3_i/2(OMEGA_2)

== system model_fully_coupled/r_double_dot_BN/r_double_dot_CN ==
  Constant : Constant  Value=F
  Gain : Gain  Gain=1/m_sc
  Out1 : Outport
  wires:
  Constant/1 -> Gain/1
  Gain/1 -> Out1/1

== system model_fully_coupled/sigma_dot_BN/Subsystem ==
  sigma_BN : Inport
  Demux : Demux  Outputs=3
  skew : MATLAB Function  TreatAsAtomicUnit=on
  "skew " : Outport
  wires:
  sigma_BN/1 -> Demux/1
  Demux/3 -> skew/3(a_3)
  Demux/2 -> skew/2(a_2)
  Demux/1 -> skew/1(a_1)
  skew/1(skew) -> "skew "/1

== system model_fully_coupled/H_sc_B/1/Subsystem ==
  Constant1 : Constant  Value=r_Bc_B
  Matrix Multiply1 : Product  Multiplication=Matrix(*)
  Out1 : Outport
  wires:
  [omega_BN_skew] -> Matrix Multiply1/1
  Constant1/1 -> Matrix Multiply1/2
  Matrix Multiply1/1 -> Out1/1

== system model_fully_coupled/H_sc_B/1/Subsystem1 ==
  1 : Inport
  Demux : Demux  Outputs=3
  skew : MATLAB Function  TreatAsAtomicUnit=on
  "skew " : Outport
  wires:
  1/1 -> Demux/1
  Demux/3 -> skew/3(a_3)
  Demux/2 -> skew/2(a_2)
  Demux/1 -> skew/1(a_1)
  skew/1(skew) -> "skew "/1

== system model_fully_coupled/H_sc_B/2/H_rw1_B ==
  I_rw1_Wc1 : Inport
  g_s_1 : Inport  Port=2
  d_1 : Inport  Port=3
  w_3_1 : Inport  Port=4
  omega_BN : Inport  Port=5
  OMEGA_1 : Inport  Port=6
  Add : Sum
  Add1 : Sum
  Matrix Multiply1 : Product  Multiplication=Matrix(*)
  Matrix Multiply2 : Product  Multiplication=Matrix(*)
  Product : Product
  Subsystem : Subsystem
  Out1 : Outport
  wires:
  Product/1 -> Add/2
  g_s_1/1 -> Product/2
  I_rw1_Wc1/1 -> Matrix Multiply1/1
  Add/1 -> Matrix Multiply1/2
  OMEGA_1/1 -> Subsystem/1(OMEGA_1), Product/1
  omega_BN/1 -> Add/1
  d_1/1 -> Subsystem/2(d_1)
  w_3_1/1 -> Subsystem/3(w_3_1)
  [r_Wc1_B_skew] -> Matrix Multiply2/1
  Subsystem/1(Out1) -> Matrix Multiply2/2
  Matrix Multiply1/1 -> Add1/1
  Add1/1 -> Out1/1
  Matrix Multiply2/1 -> Add1/2

== system model_fully_coupled/H_sc_B/2/H_rw2_B ==
  I_rw2_Wc2 : Inport
  g_s_2 : Inport  Port=2
  d_2 : Inport  Port=3
  w_3_2 : Inport  Port=4
  omega_BN : Inport  Port=5
  OMEGA_2 : Inport  Port=6
  Add : Sum
  Add1 : Sum
  Matrix Multiply1 : Product  Multiplication=Matrix(*)
  Matrix Multiply2 : Product  Multiplication=Matrix(*)
  Product : Product
  Subsystem : Subsystem
  Out1 : Outport
  wires:
  Add1/1 -> Out1/1
  OMEGA_2/1 -> Subsystem/1(OMEGA_2), Product/1
  I_rw2_Wc2/1 -> Matrix Multiply1/1
  g_s_2/1 -> Product/2
  omega_BN/1 -> Add/1
  Subsystem/1(Out1) -> Matrix Multiply2/2
  w_3_2/1 -> Subsystem/3(w_3_2)
  Product/1 -> Add/2
  Matrix Multiply2/1 -> Add1/2
  Matrix Multiply1/1 -> Add1/1
  Add/1 -> Matrix Multiply1/2
  [r_Wc2_B_skew] -> Matrix Multiply2/1
  d_2/1 -> Subsystem/2(d_2)

== system model_fully_coupled/H_sc_B/2/H_rw3_B ==
  I_rw3_Wc3 : Inport
  g_s_3 : Inport  Port=2
  d_3 : Inport  Port=3
  w_3_3 : Inport  Port=4
  omega_BN : Inport  Port=5
  OMEGA_3 : Inport  Port=6
  Add : Sum
  Add1 : Sum
  Matrix Multiply1 : Product  Multiplication=Matrix(*)
  Matrix Multiply2 : Product  Multiplication=Matrix(*)
  Product : Product
  Subsystem : Subsystem
  Out1 : Outport
  wires:
  Add1/1 -> Out1/1
  OMEGA_3/1 -> Subsystem/1(OMEGA_3), Product/1
  I_rw3_Wc3/1 -> Matrix Multiply1/1
  g_s_3/1 -> Product/2
  omega_BN/1 -> Add/1
  Subsystem/1(Out1) -> Matrix Multiply2/2
  w_3_3/1 -> Subsystem/3(w_3_3)
  Product/1 -> Add/2
  Matrix Multiply2/1 -> Add1/2
  Matrix Multiply1/1 -> Add1/1
  Add/1 -> Matrix Multiply1/2
  [r_Wc3_B_skew] -> Matrix Multiply2/1
  d_3/1 -> Subsystem/2(d_3)

== system model_fully_coupled/H_sc_B/2/I_rwi_Wci1 ==
  Out1 : Outport
  2 : Outport  Port=2
  3 : Outport  Port=3
  wires:
  [I_rw1_Wc1] -> Out1/1
  [I_rw3_Wc3] -> 3/1
  [I_rw2_Wc2] -> 2/1

== system model_fully_coupled/H_sc_B/2/Subsystem ==
  w_3_1 : Outport
  w_3_2 : Outport  Port=2
  w_3_3 : Outport  Port=3
  wires:
  [w_3_3] -> w_3_3/1
  [w_3_1] -> w_3_1/1
  [w_3_2] -> w_3_2/1

== system model_fully_coupled/H_sc_B/2/d_i ==
  d_1 : Constant  Value=d_1
  d_2 : Constant  Value=d_2
  d_3 : Constant  Value=d_3
  1 : Outport
  Out3 : Outport  Port=2
  Out2 : Outport  Port=3
  wires:
  d_3/1 -> Out3/1
  d_1/1 -> 1/1
  d_2/1 -> Out2/1

== system model_fully_coupled/H_sc_B/2/g_s_i ==
  g_s_1 : Constant  Value=g_s_1
  g_s_2 : Constant  Value=g_s_2
  g_s_3 : Constant  Value=g_s_3
  Out1 : Outport
  Out2 : Outport  Port=2
  Out3 : Outport  Port=3
  wires:
  g_s_3/1 -> Out3/1
  g_s_1/1 -> Out1/1
  g_s_2/1 -> Out2/1

== system model_fully_coupled/OMEGA_dot_i/1/1 ==
  r_double_dot_BN : Inport
  m_rw_1 : Inport  Port=2
  d_1 : Inport  Port=3
  w_3(T)_1 : Inport  Port=4
  Matrix Multiply : Product  Multiplication=Matrix(*)
  Product : Product
  Product1 : Product
  Out1 : Outport
  wires:
  Product/1 -> Product1/2
  w_3(T)_1/1 -> Product/2
  m_rw_1/1 -> Product1/1
  Product1/1 -> Matrix Multiply/1
  r_double_dot_BN/1 -> Matrix Multiply/2
  d_1/1 -> Product/1
  Matrix Multiply/1 -> Out1/1

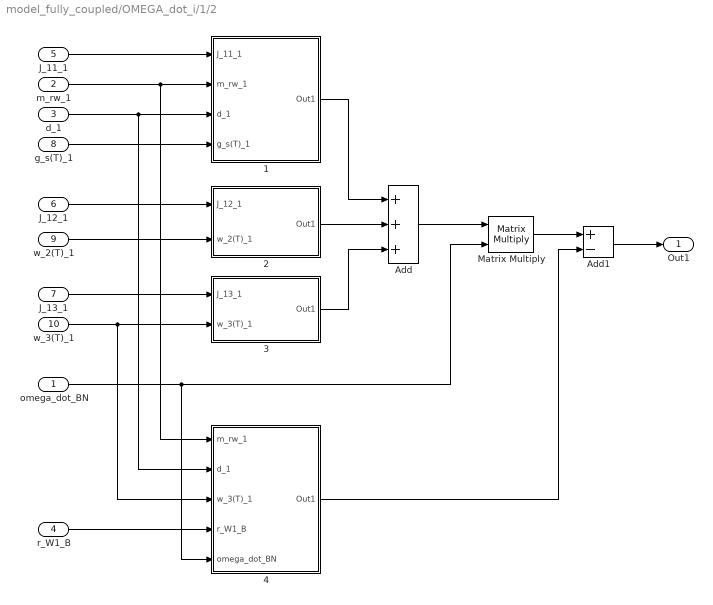
== system model_fully_coupled/OMEGA_dot_i/1/2 ==
  omega_dot_BN : Inport
  m_rw_1 : Inport  Port=2
  d_1 : Inport  Port=3
  r_W1_B : Inport  Port=4
  J_11_1 : Inport  Port=5
  J_12_1 : Inport  Port=6
  J_13_1 : Inport  Port=7
  g_s(T)_1 : Inport  Port=8
  w_2(T)_1 : Inport  Port=9
  w_3(T)_1 : Inport  Port=10
  1 : Subsystem
  2 : Subsystem
  3 : Subsystem
  4 : Subsystem
  Add : Sum  Inputs=+++
  Add1 : Sum  Inputs=+-
  Matrix Multiply : Product  Multiplication=Matrix(*)
  Out1 : Outport
  wires:
  omega_dot_BN/1 -> Matrix Multiply/2, 4/5(omega_dot_BN)
  J_12_1/1 -> 2/1(J_12_1)
  r_W1_B/1 -> 4/4(r_W1_B)
  J_13_1/1 -> 3/1(J_13_1)
  w_2(T)_1/1 -> 2/2(w_2(T)_1)
  w_3(T)_1/1 -> 4/3(w_3(T)_1), 3/2(w_3(T)_1)
  d_1/1 -> 4/2(d_1), 1/3(d_1)
  J_11_1/1 -> 1/1(J_11_1)
  m_rw_1/1 -> 4/1(m_rw_1), 1/2(m_rw_1)
  g_s(T)_1/1 -> 1/4(g_s(T)_1)
  2/1(Out1) -> Add/2
  1/1(Out1) -> Add/1
  3/1(Out1) -> Add/3
  Add/1 -> Matrix Multiply/1
  Matrix Multiply/1 -> Add1/1
  4/1(Out1) -> Add1/2
  Add1/1 -> Out1/1

== system model_fully_coupled/OMEGA_dot_i/1/3 ==
  w_w_2_1 : Inport
  w_w_3_1 : Inport  Port=2
  J_23_1 : Inport  Port=3
  Add2 : Sum  Inputs=+-
  Product1 : Product
  Product3 : Product
  Product4 : Product
  Out1 : Outport
  wires:
  Add2/1 -> Product4/2
  w_w_3_1/1 -> Product1/2, Product1/1
  Product1/1 -> Add2/1
  J_23_1/1 -> Product4/1
  w_w_2_1/1 -> Product3/2, Product3/1
  Product3/1 -> Add2/2
  Product4/1 -> Out1/1

== system model_fully_coupled/OMEGA_dot_i/1/4 ==
  w_s_1 : Inport
  w_w_2_1 : Inport  Port=2
  w_w_3_1 : Inport  Port=3
  J_12_1 : Inport  Port=4
  J_13_1 : Inport  Port=5
  Add2 : Sum  Inputs=+-
  Product1 : Product
  Product3 : Product
  Product4 : Product
  Out1 : Outport
  wires:
  J_12_1/1 -> Product1/1
  Product3/1 -> Add2/2
  J_13_1/1 -> Product3/1
  Product4/1 -> Out1/1
  Product1/1 -> Add2/1
  Add2/1 -> Product4/2
  w_s_1/1 -> Product4/1
  w_w_3_1/1 -> Product1/2
  w_w_2_1/1 -> Product3/2

== system model_fully_coupled/OMEGA_dot_i/1/5 ==
  w_w_2_1 : Inport
  w_w_3_1 : Inport  Port=2
  m_rw_1 : Inport  Port=3
  d_1 : Inport  Port=4
  J_22_1 : Inport  Port=5
  J_33_1 : Inport  Port=6
  Add2 : Sum  Inputs=+--
  Product{1,3..5} (4 alike) : Product
  Out1 : Outport
  wires:
  Product3/1 -> Add2/3
  J_33_1/1 -> Add2/2
  Product1/1 -> Product3/2
  Product4/1 -> Product5/2
  Add2/1 -> Product4/2
  Product5/1 -> Out1/1
  w_w_3_1/1 -> Product4/1
  w_w_2_1/1 -> Product5/1
  J_22_1/1 -> Add2/1
  d_1/1 -> Product1/2, Product1/1
  m_rw_1/1 -> Product3/1

== system model_fully_coupled/OMEGA_dot_i/1/6 ==
  m_rw_1 : Inport
  d_1 : Inport  Port=2
  r_W1_B : Inport  Port=3
  w_3(T)_1 : Inport  Port=4
  Matrix Multiply1 : Product  Multiplication=Matrix(*)
  Matrix Multiply2 : Product  Multiplication=Matrix(*)
  Matrix Multiply3 : Product  Multiplication=Matrix(*)
  Product1 : Product
  Product3 : Product
  Out1 : Outport
  wires:
  w_3(T)_1/1 -> Matrix Multiply3/1
  m_rw_1/1 -> Product3/1
  Product1/1 -> Product3/2
  Product3/1 -> Out1/1
  r_W1_B/1 -> Matrix Multiply1/2
  d_1/1 -> Product1/1
  Matrix Multiply3/1 -> Matrix Multiply2/1
  Matrix Multiply2/1 -> Matrix Multiply1/1
  Matrix Multiply1/1 -> Product1/2
  [omega_BN_skew] -> Matrix Multiply3/2, Matrix Multiply2/2

== system model_fully_coupled/OMEGA_dot_i/1/7 ==
  m_rw_1 : Inport
  d_1 : Inport  Port=2
  J_11_1 : Inport  Port=3
  Add1 : Sum
  Product : Product
  Product1 : Product
  Out1 : Outport
  wires:
  Product/1 -> Product1/2
  Product1/1 -> Add1/2
  d_1/1 -> Product/2, Product/1
  J_11_1/1 -> Add1/1
  Add1/1 -> Out1/1
  m_rw_1/1 -> Product1/1

== system model_fully_coupled/OMEGA_dot_i/1/Subsystem ==
  omega_BN : Inport
  omega_dot_BN : Inport  Port=2
  OMEGA_1 : Inport  Port=3
  g_s(T)_1 : Inport  Port=4
  w_2(T)_1 : Inport  Port=5
  w_3(T)_1 : Inport  Port=6
  w_s_1 : Subsystem
  w_w_2_1 : Subsystem
  w_w_3_1 : Subsystem
  1 : Outport
  2 : Outport  Port=2
  3 : Outport  Port=3
  wires:
  w_w_3_1/1(1) -> 2/1
  w_3(T)_1/1 -> w_w_3_1/4(w_3(T)_1)
  w_s_1/1(1) -> 3/1
  omega_dot_BN/1 -> w_s_1/2(omega_dot_BN), w_w_3_1/2(omega_dot_BN), w_w_2_1/2(omega_dot_BN)
  OMEGA_1/1 -> w_w_3_1/3(OMEGA_1), w_w_2_1/3(OMEGA_1)
  w_w_2_1/1(1) -> 1/1
  g_s(T)_1/1 -> w_s_1/3(g_s(T)_1)
  omega_BN/1 -> w_s_1/1(omega_BN), w_w_3_1/1(omega_BN), w_w_2_1/1(omega_BN)
  w_2(T)_1/1 -> w_w_2_1/4(w_2(T)_1)

== system model_fully_coupled/OMEGA_dot_i/2/1 ==
  r_double_dot_BN : Inport
  m_rw_2 : Inport  Port=2
  d_2 : Inport  Port=3
  w_3(T)_2 : Inport  Port=4
  Matrix Multiply : Product  Multiplication=Matrix(*)
  Product : Product
  Product1 : Product
  Out1 : Outport
  wires:
  Product/1 -> Product1/2
  w_3(T)_2/1 -> Product/2
  m_rw_2/1 -> Product1/1
  Product1/1 -> Matrix Multiply/1
  r_double_dot_BN/1 -> Matrix Multiply/2
  d_2/1 -> Product/1
  Matrix Multiply/1 -> Out1/1

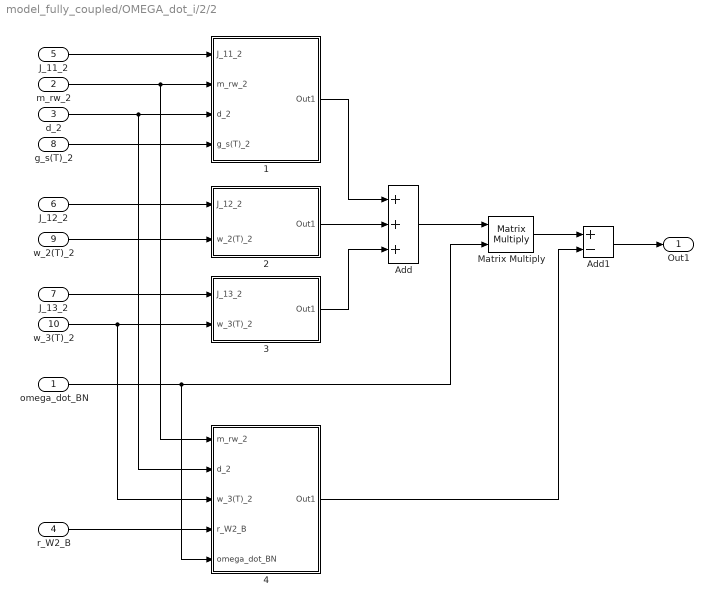
== system model_fully_coupled/OMEGA_dot_i/2/2 ==
  omega_dot_BN : Inport
  m_rw_2 : Inport  Port=2
  d_2 : Inport  Port=3
  r_W2_B : Inport  Port=4
  J_11_2 : Inport  Port=5
  J_12_2 : Inport  Port=6
  J_13_2 : Inport  Port=7
  g_s(T)_2 : Inport  Port=8
  w_2(T)_2 : Inport  Port=9
  w_3(T)_2 : Inport  Port=10
  1 : Subsystem
  2 : Subsystem
  3 : Subsystem
  4 : Subsystem
  Add : Sum  Inputs=+++
  Add1 : Sum  Inputs=+-
  Matrix Multiply : Product  Multiplication=Matrix(*)
  Out1 : Outport
  wires:
  omega_dot_BN/1 -> Matrix Multiply/2, 4/5(omega_dot_BN)
  J_12_2/1 -> 2/1(J_12_2)
  r_W2_B/1 -> 4/4(r_W2_B)
  J_13_2/1 -> 3/1(J_13_2)
  w_2(T)_2/1 -> 2/2(w_2(T)_2)
  w_3(T)_2/1 -> 4/3(w_3(T)_2), 3/2(w_3(T)_2)
  d_2/1 -> 4/2(d_2), 1/3(d_2)
  J_11_2/1 -> 1/1(J_11_2)
  m_rw_2/1 -> 4/1(m_rw_2), 1/2(m_rw_2)
  g_s(T)_2/1 -> 1/4(g_s(T)_2)
  2/1(Out1) -> Add/2
  1/1(Out1) -> Add/1
  3/1(Out1) -> Add/3
  Add/1 -> Matrix Multiply/1
  Matrix Multiply/1 -> Add1/1
  4/1(Out1) -> Add1/2
  Add1/1 -> Out1/1

== system model_fully_coupled/OMEGA_dot_i/2/3 ==
  w_w_2_2 : Inport
  w_w_3_2 : Inport  Port=2
  J_23_2 : Inport  Port=3
  Add2 : Sum  Inputs=+-
  Product1 : Product
  Product3 : Product
  Product4 : Product
  Out1 : Outport
  wires:
  Add2/1 -> Product4/2
  w_w_3_2/1 -> Product1/2, Product1/1
  Product1/1 -> Add2/1
  J_23_2/1 -> Product4/1
  w_w_2_2/1 -> Product3/2, Product3/1
  Product3/1 -> Add2/2
  Product4/1 -> Out1/1

== system model_fully_coupled/OMEGA_dot_i/2/4 ==
  w_s_2 : Inport
  w_w_2_2 : Inport  Port=2
  w_w_3_2 : Inport  Port=3
  J_12_2 : Inport  Port=4
  J_13_2 : Inport  Port=5
  Add2 : Sum  Inputs=+-
  Product1 : Product
  Product3 : Product
  Product4 : Product
  Out1 : Outport
  wires:
  J_12_2/1 -> Product1/1
  Product3/1 -> Add2/2
  J_13_2/1 -> Product3/1
  Product4/1 -> Out1/1
  Product1/1 -> Add2/1
  Add2/1 -> Product4/2
  w_s_2/1 -> Product4/1
  w_w_3_2/1 -> Product1/2
  w_w_2_2/1 -> Product3/2

== system model_fully_coupled/OMEGA_dot_i/2/5 ==
  w_w_2_2 : Inport
  w_w_3_2 : Inport  Port=2
  m_rw_2 : Inport  Port=3
  d_2 : Inport  Port=4
  J_22_2 : Inport  Port=5
  J_33_2 : Inport  Port=6
  Add2 : Sum  Inputs=+--
  Product{1,3..5} (4 alike) : Product
  Out1 : Outport
  wires:
  Product3/1 -> Add2/3
  J_33_2/1 -> Add2/2
  Product1/1 -> Product3/2
  Product4/1 -> Product5/2
  Add2/1 -> Product4/2
  Product5/1 -> Out1/1
  w_w_3_2/1 -> Product4/1
  w_w_2_2/1 -> Product5/1
  J_22_2/1 -> Add2/1
  d_2/1 -> Product1/2, Product1/1
  m_rw_2/1 -> Product3/1

== system model_fully_coupled/OMEGA_dot_i/2/6 ==
  m_rw_2 : Inport
  d_2 : Inport  Port=2
  r_W2_B : Inport  Port=3
  w_3(T)_2 : Inport  Port=4
  Matrix Multiply1 : Product  Multiplication=Matrix(*)
  Matrix Multiply2 : Product  Multiplication=Matrix(*)
  Matrix Multiply3 : Product  Multiplication=Matrix(*)
  Product1 : Product
  Product3 : Product
  Out1 : Outport
  wires:
  w_3(T)_2/1 -> Matrix Multiply3/1
  m_rw_2/1 -> Product3/1
  Product1/1 -> Product3/2
  Product3/1 -> Out1/1
  d_2/1 -> Product1/1
  Matrix Multiply3/1 -> Matrix Multiply2/1
  Matrix Multiply2/1 -> Matrix Multiply1/1
  r_W2_B/1 -> Matrix Multiply1/2
  Matrix Multiply1/1 -> Product1/2
  [omega_BN_skew] -> Matrix Multiply3/2, Matrix Multiply2/2

== system model_fully_coupled/OMEGA_dot_i/2/7 ==
  m_rw_2 : Inport
  d_2 : Inport  Port=2
  J_11_2 : Inport  Port=3
  Add1 : Sum
  Product : Product
  Product1 : Product
  Out1 : Outport
  wires:
  Product/1 -> Product1/2
  Product1/1 -> Add1/2
  d_2/1 -> Product/2, Product/1
  J_11_2/1 -> Add1/1
  Add1/1 -> Out1/1
  m_rw_2/1 -> Product1/1

== system model_fully_coupled/OMEGA_dot_i/2/Subsystem ==
  omega_BN : Inport
  omega_dot_BN : Inport  Port=2
  OMEGA_2 : Inport  Port=3
  g_s(T)_2 : Inport  Port=4
  w_2(T)_2 : Inport  Port=5
  w_3(T)_2 : Inport  Port=6
  w_s_2 : Subsystem
  w_w_2_2 : Subsystem
  w_w_3_2 : Subsystem
  1 : Outport
  2 : Outport  Port=2
  3 : Outport  Port=3
  wires:
  w_w_3_2/1(1) -> 2/1
  w_3(T)_2/1 -> w_w_3_2/4(w_3(T)_2)
  w_s_2/1(1) -> 3/1
  omega_dot_BN/1 -> w_s_2/2(omega_dot_BN), w_w_3_2/2(omega_dot_BN), w_w_2_2/2(omega_dot_BN)
  OMEGA_2/1 -> w_w_3_2/3(OMEGA_2), w_w_2_2/3(OMEGA_2)
  w_w_2_2/1(1) -> 1/1
  g_s(T)_2/1 -> w_s_2/3(g_s(T)_2)
  omega_BN/1 -> w_s_2/1(omega_BN), w_w_3_2/1(omega_BN), w_w_2_2/1(omega_BN)
  w_2(T)_2/1 -> w_w_2_2/4(w_2(T)_2)

== system model_fully_coupled/OMEGA_dot_i/3/1 ==
  r_double_dot_BN : Inport
  m_rw_3 : Inport  Port=2
  d_3 : Inport  Port=3
  w_3(T)_3 : Inport  Port=4
  Matrix Multiply : Product  Multiplication=Matrix(*)
  Product : Product
  Product1 : Product
  Out1 : Outport
  wires:
  Product/1 -> Product1/2
  w_3(T)_3/1 -> Product/2
  m_rw_3/1 -> Product1/1
  Product1/1 -> Matrix Multiply/1
  r_double_dot_BN/1 -> Matrix Multiply/2
  d_3/1 -> Product/1
  Matrix Multiply/1 -> Out1/1

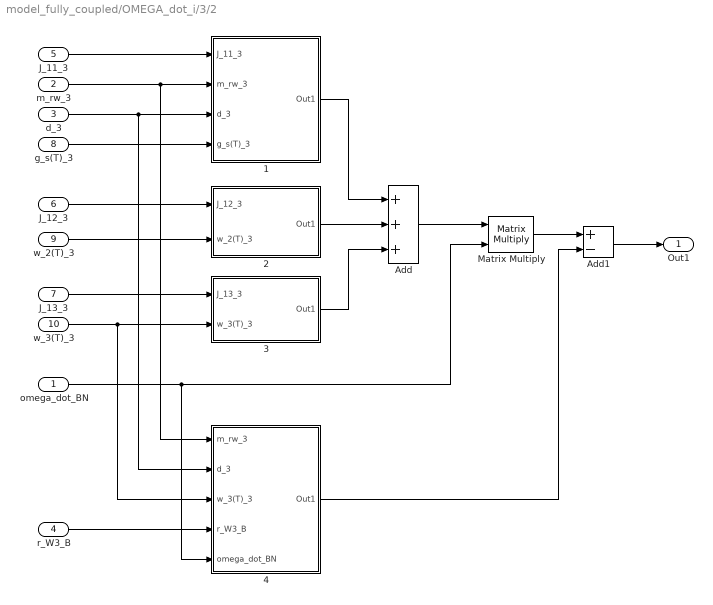
== system model_fully_coupled/OMEGA_dot_i/3/2 ==
  omega_dot_BN : Inport
  m_rw_3 : Inport  Port=2
  d_3 : Inport  Port=3
  r_W3_B : Inport  Port=4
  J_11_3 : Inport  Port=5
  J_12_3 : Inport  Port=6
  J_13_3 : Inport  Port=7
  g_s(T)_3 : Inport  Port=8
  w_2(T)_3 : Inport  Port=9
  w_3(T)_3 : Inport  Port=10
  1 : Subsystem
  2 : Subsystem
  3 : Subsystem
  4 : Subsystem
  Add : Sum  Inputs=+++
  Add1 : Sum  Inputs=+-
  Matrix Multiply : Product  Multiplication=Matrix(*)
  Out1 : Outport
  wires:
  omega_dot_BN/1 -> Matrix Multiply/2, 4/5(omega_dot_BN)
  J_12_3/1 -> 2/1(J_12_3)
  r_W3_B/1 -> 4/4(r_W3_B)
  J_13_3/1 -> 3/1(J_13_3)
  w_2(T)_3/1 -> 2/2(w_2(T)_3)
  w_3(T)_3/1 -> 4/3(w_3(T)_3), 3/2(w_3(T)_3)
  d_3/1 -> 4/2(d_3), 1/3(d_3)
  J_11_3/1 -> 1/1(J_11_3)
  m_rw_3/1 -> 4/1(m_rw_3), 1/2(m_rw_3)
  g_s(T)_3/1 -> 1/4(g_s(T)_3)
  2/1(Out1) -> Add/2
  1/1(Out1) -> Add/1
  3/1(Out1) -> Add/3
  Add/1 -> Matrix Multiply/1
  Matrix Multiply/1 -> Add1/1
  4/1(Out1) -> Add1/2
  Add1/1 -> Out1/1

== system model_fully_coupled/OMEGA_dot_i/3/3 ==
  w_w_2_3 : Inport
  w_w_3_3 : Inport  Port=2
  J_23_3 : Inport  Port=3
  Add2 : Sum  Inputs=+-
  Product1 : Product
  Product3 : Product
  Product4 : Product
  Out1 : Outport
  wires:
  Add2/1 -> Product4/2
  w_w_3_3/1 -> Product1/2, Product1/1
  Product1/1 -> Add2/1
  J_23_3/1 -> Product4/1
  w_w_2_3/1 -> Product3/2, Product3/1
  Product3/1 -> Add2/2
  Product4/1 -> Out1/1

== system model_fully_coupled/OMEGA_dot_i/3/4 ==
  w_s_3 : Inport
  w_w_2_3 : Inport  Port=2
  w_w_3_3 : Inport  Port=3
  J_12_3 : Inport  Port=4
  J_13_3 : Inport  Port=5
  Add2 : Sum  Inputs=+-
  Product1 : Product
  Product3 : Product
  Product4 : Product
  Out1 : Outport
  wires:
  J_12_3/1 -> Product1/1
  Product3/1 -> Add2/2
  J_13_3/1 -> Product3/1
  Product4/1 -> Out1/1
  Product1/1 -> Add2/1
  Add2/1 -> Product4/2
  w_s_3/1 -> Product4/1
  w_w_3_3/1 -> Product1/2
  w_w_2_3/1 -> Product3/2

== system model_fully_coupled/OMEGA_dot_i/3/5 ==
  w_w_2_3 : Inport
  w_w_3_3 : Inport  Port=2
  m_rw_3 : Inport  Port=3
  d_3 : Inport  Port=4
  J_22_3 : Inport  Port=5
  J_33_3 : Inport  Port=6
  Add2 : Sum  Inputs=+--
  Product{1,3..5} (4 alike) : Product
  Out1 : Outport
  wires:
  Product3/1 -> Add2/3
  J_33_3/1 -> Add2/2
  Product1/1 -> Product3/2
  Product4/1 -> Product5/2
  Add2/1 -> Product4/2
  Product5/1 -> Out1/1
  w_w_3_3/1 -> Product4/1
  w_w_2_3/1 -> Product5/1
  J_22_3/1 -> Add2/1
  d_3/1 -> Product1/2, Product1/1
  m_rw_3/1 -> Product3/1

== system model_fully_coupled/OMEGA_dot_i/3/6 ==
  m_rw_3 : Inport
  d_3 : Inport  Port=2
  r_W3_B : Inport  Port=3
  w_3(T)_3 : Inport  Port=4
  Matrix Multiply1 : Product  Multiplication=Matrix(*)
  Matrix Multiply2 : Product  Multiplication=Matrix(*)
  Matrix Multiply3 : Product  Multiplication=Matrix(*)
  Product1 : Product
  Product3 : Product
  Out1 : Outport
  wires:
  w_3(T)_3/1 -> Matrix Multiply3/1
  m_rw_3/1 -> Product3/1
  Product1/1 -> Product3/2
  Product3/1 -> Out1/1
  d_3/1 -> Product1/1
  Matrix Multiply3/1 -> Matrix Multiply2/1
  Matrix Multiply2/1 -> Matrix Multiply1/1
  r_W3_B/1 -> Matrix Multiply1/2
  Matrix Multiply1/1 -> Product1/2
  [omega_BN_skew] -> Matrix Multiply3/2, Matrix Multiply2/2

== system model_fully_coupled/OMEGA_dot_i/3/7 ==
  m_rw_3 : Inport
  d_3 : Inport  Port=2
  J_11_3 : Inport  Port=3
  Add1 : Sum
  Product : Product
  Product1 : Product
  Out1 : Outport
  wires:
  Product/1 -> Product1/2
  Product1/1 -> Add1/2
  d_3/1 -> Product/2, Product/1
  J_11_3/1 -> Add1/1
  Add1/1 -> Out1/1
  m_rw_3/1 -> Product1/1

== system model_fully_coupled/OMEGA_dot_i/3/Subsystem ==
  omega_BN : Inport
  omega_dot_BN : Inport  Port=2
  OMEGA_3 : Inport  Port=3
  g_s(T)_3 : Inport  Port=4
  w_2(T)_3 : Inport  Port=5
  w_3(T)_3 : Inport  Port=6
  w_s_3 : Subsystem
  w_w_2_3 : Subsystem
  w_w_3_3 : Subsystem
  1 : Outport
  2 : Outport  Port=2
  3 : Outport  Port=3
  wires:
  w_w_3_3/1(1) -> 2/1
  w_3(T)_3/1 -> w_w_3_3/4(w_3(T)_3)
  w_s_3/1(1) -> 3/1
  omega_dot_BN/1 -> w_s_3/2(omega_dot_BN), w_w_3_3/2(omega_dot_BN), w_w_2_3/2(omega_dot_BN)
  OMEGA_3/1 -> w_w_3_3/3(OMEGA_3), w_w_2_3/3(OMEGA_3)
  w_w_2_3/1(1) -> 1/1
  g_s(T)_3/1 -> w_s_3/3(g_s(T)_3)
  omega_BN/1 -> w_s_3/1(omega_BN), w_w_3_3/1(omega_BN), w_w_2_3/1(omega_BN)
  w_2(T)_3/1 -> w_w_2_3/4(w_2(T)_3)

== system model_fully_coupled/omega_dot_BN/2 /Subsystem1 ==
  1 : Inport
  Demux : Demux  Outputs=3
  skew : MATLAB Function  TreatAsAtomicUnit=on
  "skew " : Outport
  wires:
  1/1 -> Demux/1
  Demux/3 -> skew/3(a_3)
  Demux/2 -> skew/2(a_2)
  Demux/1 -> skew/1(a_1)
  skew/1(skew) -> "skew "/1

== system model_fully_coupled/omega_dot_BN/3/I_sc_B ==
  OMEGA_1 : Inport
  OMEGA_2 : Inport  Port=2
  OMEGA_3 : Inport  Port=3
  Add : Sum
  I_hub_B : Subsystem
  I_rwi_B : Subsystem
  I_sc_B : Outport
  wires:
  I_rwi_B/1(Out1) -> Add/2
  Add/1 -> I_sc_B/1
  I_hub_B/1(Out1) -> Add/1
  OMEGA_1/1 -> I_rwi_B/1(OMEGA_1)
  OMEGA_2/1 -> I_rwi_B/2(OMEGA_2)
  OMEGA_3/1 -> I_rwi_B/3(OMEGA_3)

== system model_fully_coupled/omega_dot_BN/3/I_sc_B' ==
  Add : Sum  Inputs=+++
  I_rw1_B' : Subsystem
  I_rw2_B' : Subsystem
  I_rw3_B' : Subsystem
  I_rwi_Wci' : Subsystem
  m_rw_i : Subsystem
  Out1 : Outport
  wires:
  m_rw_i/2(Out2) -> I_rw2_B'/2(m_rw_2)
  m_rw_i/3(Out3) -> I_rw3_B'/2(m_rw_3)
  I_rw1_B'/1(Out1) -> Add/1
  m_rw_i/1(Out1) -> I_rw1_B'/2(m_rw_1)
  I_rwi_Wci'/3(3) -> I_rw3_B'/1(I_rw3_Wc3')
  I_rw2_B'/1(Out2) -> Add/2
  Add/1 -> Out1/1
  I_rwi_Wci'/1(1) -> I_rw1_B'/1(I_rw1_Wc1')
  I_rw3_B'/1(Out3) -> Add/3
  I_rwi_Wci'/2(2) -> I_rw2_B'/1(I_rw2_Wc2')

== system model_fully_coupled/omega_dot_BN/4/I_rwi_Wci ==
  Out1 : Outport
  Out2 : Outport  Port=2
  Out3 : Outport  Port=3
  wires:
  [I_rw1_Wc1] -> Out1/1
  [I_rw3_Wc3] -> Out3/1
  [I_rw2_Wc2] -> Out2/1

== system model_fully_coupled/omega_dot_BN/4/g_s_i ==
  g_s_1 : Constant  Value=g_s_1
  g_s_2 : Constant  Value=g_s_2
  g_s_3 : Constant  Value=g_s_3
  Out1 : Outport
  Out2 : Outport  Port=2
  Out3 : Outport  Port=3
  wires:
  g_s_3/1 -> Out3/1
  g_s_1/1 -> Out1/1
  g_s_2/1 -> Out2/1

== system model_fully_coupled/omega_dot_BN/5/I_rwi_Wci' ==
  Out1 : Outport
  Out2 : Outport  Port=2
  Out3 : Outport  Port=3
  wires:
  [I_rw1_Wc1_] -> Out1/1
  [I_rw3_Wc3_] -> Out3/1
  [I_rw2_Wc2_] -> Out2/1

== system model_fully_coupled/omega_dot_BN/5/g_s_i ==
  g_s_1 : Constant  Value=g_s_1
  g_s_2 : Constant  Value=g_s_2
  g_s_3 : Constant  Value=g_s_3
  Out1 : Outport
  Out2 : Outport  Port=2
  Out3 : Outport  Port=3
  wires:
  g_s_3/1 -> Out3/1
  g_s_1/1 -> Out1/1
  g_s_2/1 -> Out2/1
